simulink model "Follower"  (R2018a)
settings: Solver=FixedStepAuto  StartTime=0.0  StopTime=300  FixedStep=0.1  RelTol=1e-3
libraries: simulink x1
settings Model: Creator=wangluo  LastModifiedBy=wangluo

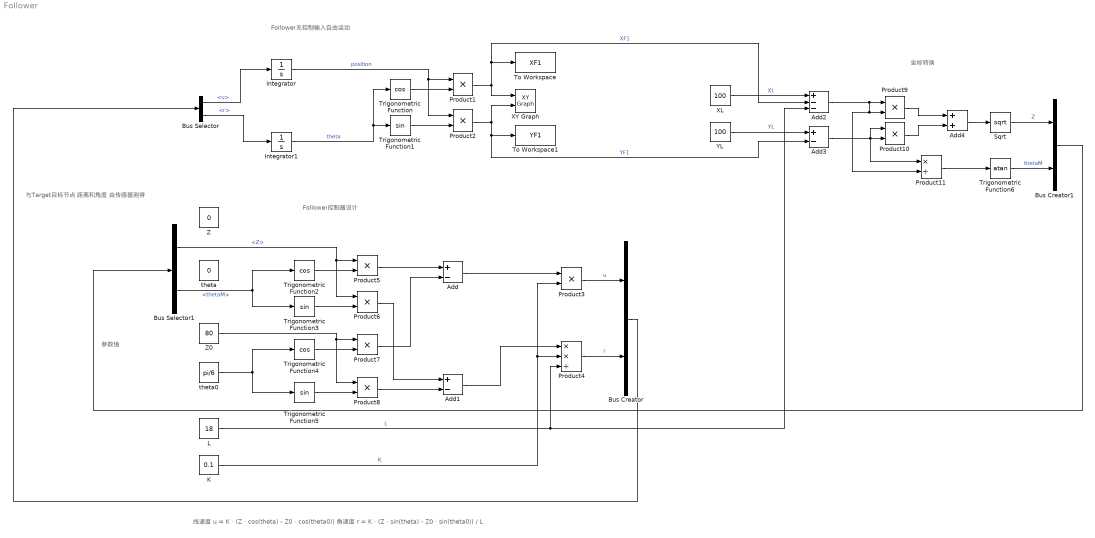
== system Follower ==
  note: Follower无控制输入自由运动
  note: Follower控制器设计
  note: 与Target目标节点
      | 距离和角度
      | 由传感器测得
  note: 参数值
  note: 线速度 u = K · (Z · cos(theta) - Z0 · cos(theta0))
      | 角速度 r = K · (Z · sin(theta) - Z0 · sin(theta0)) / L
  note: 坐标转换
  Add : Sum  Inputs=+-
  Add1 : Sum  Inputs=+-
  Add2 : Sum  Inputs=+--
  Add3 : Sum  Inputs=+-
  Add4 : Sum
  Bus Creator : BusCreator  Inputs=2
  Bus Creator1 : BusCreator  Inputs=2
  Bus Selector : BusSelector  OutputSignals=u,r
  Bus Selector1 : BusSelector  OutputSignals=Z,thetaM
  Integrator : Integrator
  Integrator1 : Integrator
  K : Constant  Value=0.1
  L : Constant  Value=18
  Product{1..3,5..10} (9 alike) : Product
  Product11 : Product  Inputs=*/
  Product4 : Product  Inputs=**/
  Sqrt : Sqrt  SaturateOnIntegerOverflow=on
  To Workspace : ToWorkspace  VariableName=XF1  SaveFormat=Timeseries  SampleTime=-1
  To Workspace1 : ToWorkspace  VariableName=YF1  SaveFormat=Timeseries  SampleTime=-1
  Trigonometric Function : Trigonometry  Operator=cos
  Trigonometric Function1 : Trigonometry
  Trigonometric Function2 : Trigonometry  Operator=cos
  Trigonometric Function3 : Trigonometry
  Trigonometric Function4 : Trigonometry  Operator=cos
  Trigonometric Function5 : Trigonometry
  Trigonometric Function6 : Trigonometry  Operator=atan
  XL : Constant  Value=100
  XY Graph : simulink/Sinks/XY Graph  xmin=-200  xmax=500  ymin=-200  ymax=500  st=-1
  YL : Constant  Value=100
  Z : Constant  Value=0
  Z0 : Constant  Value=80
  theta : Constant  Value=0
  theta0 : Constant  Value=pi/6
  wires:
  Integrator1/1 -> Trigonometric Function1/1, Trigonometric Function/1  "theta"
  Product1/1 -> Add2/2, To Workspace/1, XY Graph/1  "XF1"
  Product2/1 -> XY Graph/2, Add3/2, To Workspace1/1  "YF1"
  Trigonometric Function/1 -> Product1/2
  Trigonometric Function1/1 -> Product2/2
  Integrator/1 -> Product2/1, Product1/1  "position"
  Product4/1 -> Bus Creator/2  "r"
  Product3/1 -> Bus Creator/1  "u"
  Bus Creator/1 -> Bus Selector/1
  Bus Selector/1 -> Integrator/1  "<u>"
  Bus Selector/2 -> Integrator1/1  "<r>"
  Bus Selector1/2 -> Trigonometric Function3/1, Trigonometric Function2/1  "<thetaM>"
  theta0/1 -> Trigonometric Function5/1, Trigonometric Function4/1
  Trigonometric Function2/1 -> Product5/2
  Trigonometric Function3/1 -> Product6/2
  Bus Selector1/1 -> Product6/1, Product5/1  "<Z>"
  Trigonometric Function4/1 -> Product7/2
  Trigonometric Function5/1 -> Product8/2
  Z0/1 -> Product8/1, Product7/1
  Product5/1 -> Add/1
  Product7/1 -> Add/2
  Product8/1 -> Add1/2
  Product6/1 -> Add1/1
  Add/1 -> Product3/1
  K/1 -> Product3/2, Product4/2  "K"
  Add1/1 -> Product4/1
  L/1 -> Add2/3, Product4/3  "L"
  YL/1 -> Add3/1  "YL"
  XL/1 -> Add2/1  "XL"
  Sqrt/1 -> Bus Creator1/1  "Z"
  Add2/1 -> Product11/2, Product9/2, Product9/1
  Add3/1 -> Product11/1, Product10/2, Product10/1
  Product9/1 -> Add4/1
  Product10/1 -> Add4/2
  Add4/1 -> Sqrt/1
  Trigonometric Function6/1 -> Bus Creator1/2  "thetaM"
  Product11/1 -> Trigonometric Function6/1
  Bus Creator1/1 -> Bus Selector1/1
